simulink library "slrthdlutillib"  (R2022a)
settings: Solver=VariableStepAuto  StartTime=0.0  StopTime=10.0  RelTol=1e-3
libraries: hdlsllib x5, simulink x2
settings Model: Creator=chrisz  LastModifiedBy=chrisz

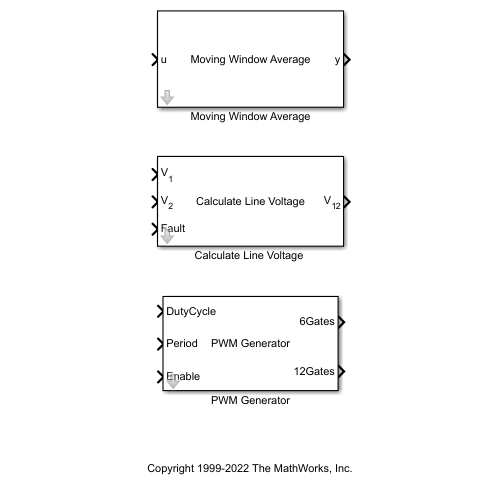
[thumbnail: Simulink's stored preview of the top-level diagram]
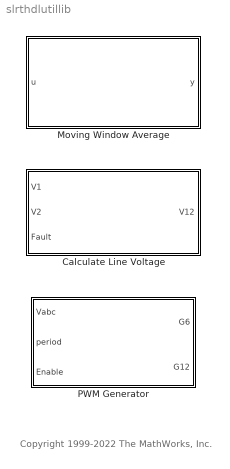
== system slrthdlutillib ==
  note: Copyright 1999-2022 The MathWorks, Inc.
  "Calculate Line Voltage " : Subsystem  mask(Calculate Line Voltage){}
      mask help: This block calculates the line voltage between V1 and V2. A fault occurs on a line by assigning value greater than zero to the corresponding port.
      mask Display:
      | disp('Calculate Line Voltage');
      | port_label('input', 1, 'V_1','texmode','on');
      | port_label('input', 2, 'V_2','texmode','on');
      | port_label('input', 3, 'Fault');
      | port_label('output', 1, 'V_1_2','texmode','on');
  Moving Window Average : Subsystem  mask(Moving Window Average){sample_time=5e-9, window_size=1e-6}
      mask prompts: sample_time "Base Sample Time (s)"; window_size "Window Size (s)"
      mask help:
      | This block implements a moving window average algorithm, that converts a boolean signal, to a duty ratio. It's resolution is set by the clock rate, and the width of the window is set by window size.  For example, if we are implementing a moving window average on an FPGA running at 200Mhz, but want that signal to feed a model running at 1 Mhz, the clock time step would be 5e-9 (1/200000000) while the window size would be 1e-6. This would effectively calculate an average every 200 FPGA clock cycles.
      |
      | This block was specifically designed to run on FPGA's utilizing subcycle averaging.
      mask init:
      | oversampling = round(window_size/sample_time);
      mask Display:
      | disp('Moving Window Average');
      | port_label('input', 1, 'u');
      | port_label('output', 1, 'y');
  PWM Generator : Subsystem  mask(PWM Generator){}
      mask help: HDL coder compatible implementation of PWM generator. This model simulates FPGA clock level operations and is not suited for desktop simulation other than for validating the real-time model is accurate. It should primarily be used when generating HDL for real-time systems. Use standard blocks for desktop simulation.
      mask Display:
      | disp('PWM Generator')
      | port_label('input', 1, 'DutyCycle')
      | port_label('input', 2, 'Period')
      | port_label('input', 3, 'Enable')
      | port_label('output', 1, '6Gates')
      | port_label('output', 2, '12Gates')

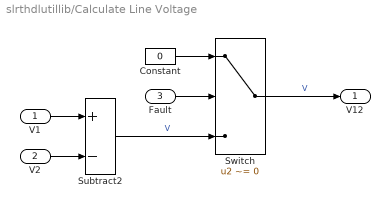
== system slrthdlutillib/Calculate Line Voltage  ==
  V1 : Inport
  V2 : Inport  Port=2
  Fault : Inport  Port=3
  Constant : Constant  Value=0  OutDataTypeStr=single  SampleTime=-1
  Subtract2 : Sum  Inputs=+-
  Switch : Switch  Criteria=u2 ~= 0  SaturateOnIntegerOverflow=off  InputSameDT=off
  V12 : Outport  VectorParamsAs1DForOutWhenUnconnected=off
  wires:
  V2/1 -> Subtract2/2
  V1/1 -> Subtract2/1
  Subtract2/1 -> Switch/3  "V"
  Fault/1 -> Switch/2
  Switch/1 -> V12/1  "V"
  Constant/1 -> Switch/1

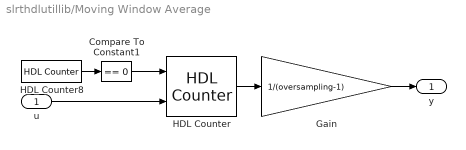
== system slrthdlutillib/Moving Window Average ==
  u : Inport  OutDataTypeStr=boolean
  Compare To Constant1 : simulink/Logic and Bit Operations/Compare To Constant  relop===  const=0  OutDataTypeStr=boolean
  Gain : Gain  Gain=1/(oversampling-1)  OutDataTypeStr=fixdt(0,18,17)  RndMeth=Zero  SaturateOnIntegerOverflow=on
  HDL Counter : hdlsllib/Sources/HDL Counter  CountType=Count limited  CountInit=0  CountStep=1  CountMax=oversampling-1  CountFromType=Initial value  CountFrom=0  CountResetPort=on  CountLoadPort=off  CountEnbPort=on  CountDirPort=off  CountHitOutputPort=off  CountDataType=Unsigned  CountWordLen=12  CountFracLen=0  CountSampTime=1
  HDL Counter8 : hdlsllib/Sources/HDL Counter  CountType=Count limited  CountInit=0  CountStep=1  CountMax=oversampling-1  CountFromType=Initial value  CountFrom=0  CountResetPort=off  CountLoadPort=off  CountEnbPort=off  CountDirPort=off  CountHitOutputPort=off  CountDataType=Unsigned  CountWordLen=12  CountFracLen=0  CountSampTime=sample_time
  y : Outport
  wires:
  Gain/1 -> y/1
  HDL Counter8/1 -> Compare To Constant1/1
  Compare To Constant1/1 -> HDL Counter/1
  HDL Counter/1 -> Gain/1
  u/1 -> HDL Counter/2

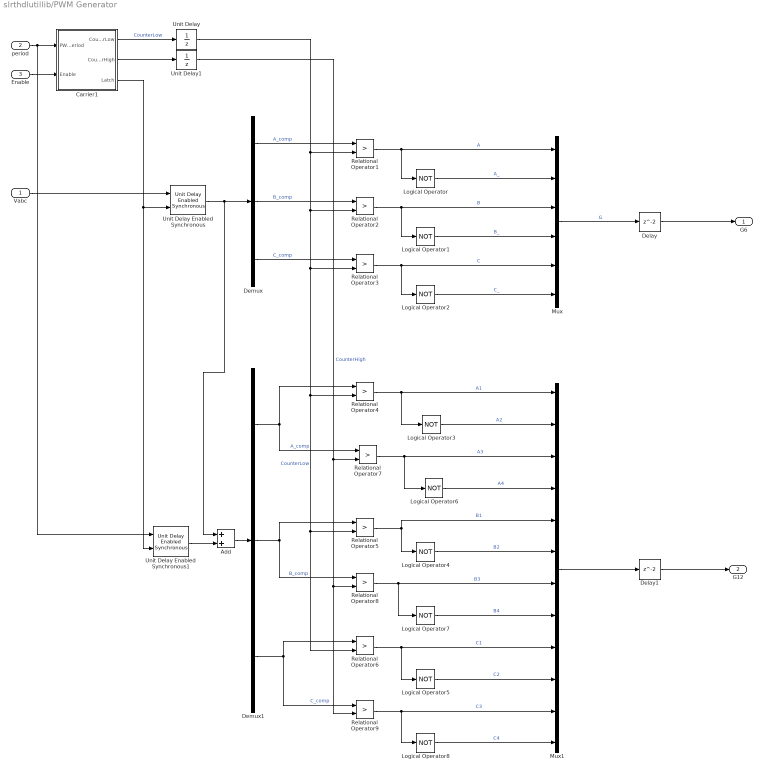
== system slrthdlutillib/PWM Generator ==
  Vabc : Inport
  period : Inport  Port=2
  Enable : Inport  Port=3
  Add : Sum
  Carrier1 : Subsystem
  Delay : Delay
  Delay1 : Delay
  Demux : Demux  Outputs=3
  Demux1 : Demux  Outputs=3
  Logical Operator{,1..8} (9 alike) : Logic  Operator=NOT  AllPortsSameDT=off  OutDataTypeStr=boolean
  Mux : Mux  Inputs=6
  Mux1 : Mux  Inputs=12
  Relational Operator{1..9} (9 alike) : RelationalOperator  Operator=>  OutDataTypeStr=boolean  InputSameDT=off
  Unit Delay : UnitDelay  SampleTime=-1  HasFrameUpgradeWarning=on
  Unit Delay Enabled Synchronous : hdlsllib/Discrete/Unit Delay Enabled Synchronous  InitialCondition=0.0  SampleTime=-1
      settings: SourceProductName=HDL Coder
  Unit Delay Enabled Synchronous1 : hdlsllib/Discrete/Unit Delay Enabled Synchronous  InitialCondition=0.0  SampleTime=-1
      settings: SourceProductName=HDL Coder
  Unit Delay1 : UnitDelay  SampleTime=-1  HasFrameUpgradeWarning=on
  G6 : Outport  VectorParamsAs1DForOutWhenUnconnected=off
  G12 : Outport  Port=2  VectorParamsAs1DForOutWhenUnconnected=off
  wires:
  Demux/2 -> Relational Operator2/1  "B_comp"
  Logical Operator2/1 -> Mux/6  "C_"
  Relational Operator3/1 -> Mux/5, Logical Operator2/1  "C"
  Logical Operator/1 -> Mux/2  "A_"
  Vabc/1 -> Unit Delay Enabled Synchronous/1
  Logical Operator1/1 -> Mux/4  "B_"
  Unit Delay/1 -> Relational Operator1/2, Relational Operator5/2, Relational Operator6/2, Relational Operator4/2, Relational Operator3/2, Relational Operator2/2  "CounterLow"
  Demux/1 -> Relational Operator1/1  "A_comp"
  Demux/3 -> Relational Operator3/1  "C_comp"
  Relational Operator1/1 -> Logical Operator/1, Mux/1  "A"
  Relational Operator2/1 -> Mux/3, Logical Operator1/1  "B"
  Carrier1/3(Latch) -> Unit Delay Enabled Synchronous1/2, Unit Delay Enabled Synchronous/2
  Unit Delay Enabled Synchronous/1 -> Add/1, Demux/1
  Carrier1/1(CounterLow) -> Unit Delay/1  "CounterLow"
  Enable/1 -> Carrier1/2(Enable)
  Mux/1 -> Delay/1  "G"
  Delay/1 -> G6/1
  Mux1/1 -> Delay1/1
  Delay1/1 -> G12/1
  Relational Operator5/1 -> Mux1/5, Logical Operator4/1  "B1"
  Relational Operator6/1 -> Mux1/9, Logical Operator5/1  "C1"
  Relational Operator4/1 -> Mux1/1, Logical Operator3/1  "A1"
  Logical Operator3/1 -> Mux1/2  "A2"
  Relational Operator7/1 -> Mux1/3, Logical Operator6/1  "A3"
  Logical Operator6/1 -> Mux1/4  "A4"
  Demux1/1 -> Relational Operator7/1, Relational Operator4/1  "A_comp"
  Demux1/2 -> Relational Operator8/1, Relational Operator5/1  "B_comp"
  Logical Operator4/1 -> Mux1/6  "B2"
  Relational Operator8/1 -> Logical Operator7/1, Mux1/7  "B3"
  Logical Operator7/1 -> Mux1/8  "B4"
  Demux1/3 -> Relational Operator9/1, Relational Operator6/1  "C_comp"
  Logical Operator5/1 -> Mux1/10  "C2"
  Relational Operator9/1 -> Mux1/11, Logical Operator8/1  "C3"
  Logical Operator8/1 -> Mux1/12  "C4"
  Add/1 -> Demux1/1
  period/1 -> Unit Delay Enabled Synchronous1/1, Carrier1/1(PWM Period)
  Unit Delay Enabled Synchronous1/1 -> Add/2
  Carrier1/2(CounterHigh) -> Unit Delay1/1
  Unit Delay1/1 -> Relational Operator9/2, Relational Operator8/2, Relational Operator7/2  "CounterHigh"

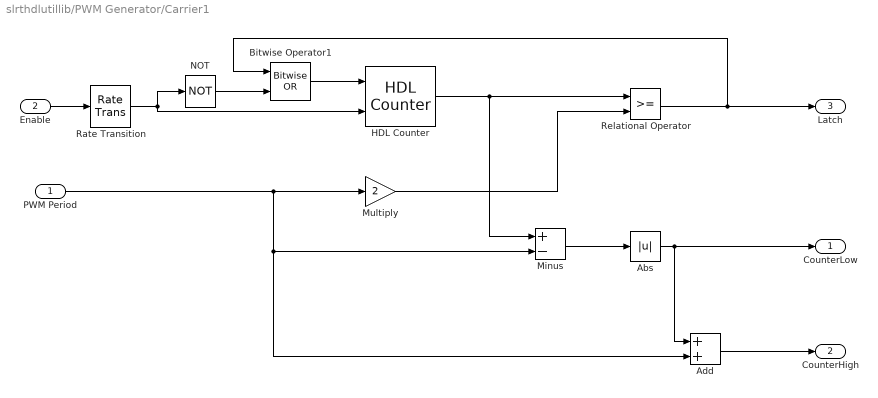
== system slrthdlutillib/PWM Generator/Carrier1 ==
  PWM Period : Inport  OutDataTypeStr=uint32  PortDimensions=1
  Enable : Inport  Port=2  OutDataTypeStr=boolean  PortDimensions=1
  Abs : Abs  OutDataTypeStr=uint32  SaturateOnIntegerOverflow=off
  Add : Sum
  Bitwise Operator1 : simulink/Logic and Bit Operations/Bitwise Operator  logicop=OR  UseBitMask=off  NumInputPorts=2  BitMask=bin2dec('11011001')  BitMaskRealWorld=Stored Integer
  HDL Counter : hdlsllib/Sources/HDL Counter  CountType=Free running  CountInit=0  CountStep=1  CountMax=25  CountFromType=Initial value  CountFrom=0  CountResetPort=on  CountLoadPort=off  CountEnbPort=on  CountDirPort=off  CountHitOutputPort=off  CountDataType=Unsigned  CountWordLen=32  CountFracLen=0  CountSampTime=1
  Minus : Sum  Inputs=+-  OutDataTypeStr=int32
  Multiply : Gain  Gain=2  OutDataTypeStr=uint32
  NOT : Logic  Operator=NOT  AllPortsSameDT=off  OutDataTypeStr=boolean
  Rate Transition : RateTransition
  Relational Operator : RelationalOperator  OutDataTypeStr=boolean  InputSameDT=off
  CounterLow : Outport  VectorParamsAs1DForOutWhenUnconnected=off
  CounterHigh : Outport  Port=2  VectorParamsAs1DForOutWhenUnconnected=off
  Latch : Outport  Port=3
  wires:
  Rate Transition/1 -> NOT/1, HDL Counter/2
  HDL Counter/1 -> Relational Operator/1, Minus/1
  Minus/1 -> Abs/1
  Abs/1 -> Add/1, CounterLow/1
  Multiply/1 -> Relational Operator/2
  Relational Operator/1 -> Bitwise Operator1/1, Latch/1
  NOT/1 -> Bitwise Operator1/2
  Bitwise Operator1/1 -> HDL Counter/1
  Enable/1 -> Rate Transition/1
  PWM Period/1 -> Multiply/1, Add/2, Minus/2
  Add/1 -> CounterHigh/1
